simulink model "start_process_2018a"  (R2018a)
settings: Solver=FixedStepAuto  StartTime=0.0  StopTime=0.001  RelTol=1e-3
values from neighbouring files (symbols this model uses):
  trigger = true    [final_test.m]    (also in main_file.m; vel_measurement_final.m)
  velo = v_m * 1000    [final_test.m]
libraries: TcAdsLib x4
settings Model: Creator=chijiang  LastModifiedBy=chduan
settings OptimizationCC: LocalBlockOutputs=off
settings SFSimCC: SimUseLocalCustomCode=on
settings RTWCC: SystemTargetFile=TwinCAT.tlc  MakeCommand=make_tct  TemplateMakefile=tct_msbuild.tmf  Description=TwinCAT Target  GenerateReport=on  RTWUseLocalCustomCode=on  TargetLang=C++
settings STFCustomTargetCC: TargetLangStandard=C++03 (ISO)  CompOptLevelCompliant=on  MATLABClassNameForMDSCustomization=Simulink.SoftwareTarget.TargetSpecificTriggerConfigurationBase  SystemTargetFile=TwinCAT.tlc

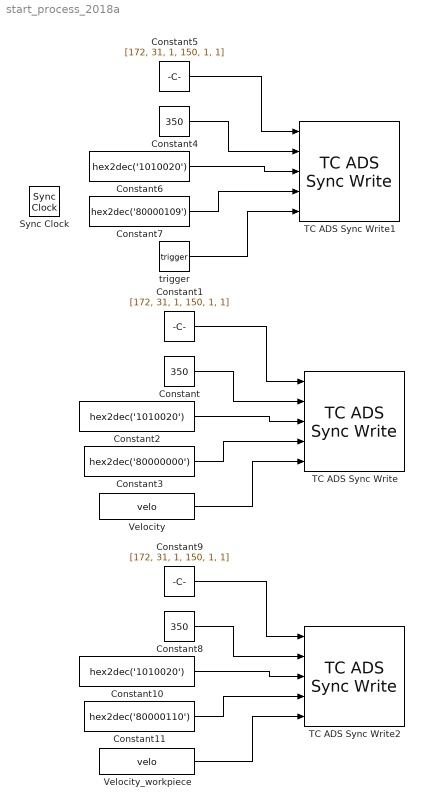
== system start_process_2018a ==
  Constant : Constant  Value=350  OutDataTypeStr=uint16
  Constant1 : Constant  Value=[172, 31, 1, 150, 1, 1]  OutDataTypeStr=uint8
  Constant10 : Constant  Value=hex2dec('1010020')  OutDataTypeStr=uint32
  Constant11 : Constant  Value=hex2dec('80000110')  OutDataTypeStr=uint32
  Constant2 : Constant  Value=hex2dec('1010020')  OutDataTypeStr=uint32
  Constant3 : Constant  Value=hex2dec('80000000')  OutDataTypeStr=uint32
  Constant4 : Constant  Value=350  OutDataTypeStr=uint16
  Constant5 : Constant  Value=[172, 31, 1, 150, 1, 1]  OutDataTypeStr=uint8
  Constant6 : Constant  Value=hex2dec('1010020')  OutDataTypeStr=uint32
  Constant7 : Constant  Value=hex2dec('80000109')  OutDataTypeStr=uint32
  Constant8 : Constant  Value=350  OutDataTypeStr=uint16
  Constant9 : Constant  Value=[172, 31, 1, 150, 1, 1]  OutDataTypeStr=uint8
  Sync Clock : TcAdsLib/Utilities/Sync Clock  OutputPortSelect=None  InputPortSelect=None
      settings: SourceProductName=Beckhoff TwinCAT ADS Interface
  TC ADS Sync Write : TcAdsLib/Synchronous/TC ADS Sync Write  SampleTime=-1  AbortSimulationOnAdsError=off  WriteDataType=double  WriteDataDim=1  WriteDataColToRowMajor=on  AdsTimeout=1  DirectFeedThrough=off  CreateSignalLabels=on  CodeGenConnectType=DataArea (OutputSrc)
      settings: SourceProductName=Beckhoff TwinCAT ADS Interface
  TC ADS Sync Write1 : TcAdsLib/Synchronous/TC ADS Sync Write  SampleTime=-1  AbortSimulationOnAdsError=off  WriteDataType=boolean  WriteDataDim=1  WriteDataColToRowMajor=on  AdsTimeout=1  DirectFeedThrough=off  CreateSignalLabels=on  CodeGenConnectType=DataArea (OutputSrc)
      settings: SourceProductName=Beckhoff TwinCAT ADS Interface
  TC ADS Sync Write2 : TcAdsLib/Synchronous/TC ADS Sync Write  SampleTime=-1  AbortSimulationOnAdsError=off  WriteDataType=double  WriteDataDim=1  WriteDataColToRowMajor=on  AdsTimeout=1  DirectFeedThrough=off  CreateSignalLabels=on  CodeGenConnectType=DataArea (OutputSrc)
      settings: SourceProductName=Beckhoff TwinCAT ADS Interface
  Velocity : Constant  Value=velo
  Velocity_workpiece : Constant  Value=velo
  trigger : Constant  Value=trigger  OutDataTypeStr=boolean
  wires:
  Constant/1 -> TC ADS Sync Write/2
  Constant2/1 -> TC ADS Sync Write/3
  Constant1/1 -> TC ADS Sync Write/1
  Velocity/1 -> TC ADS Sync Write/5
  Constant3/1 -> TC ADS Sync Write/4
  Constant7/1 -> TC ADS Sync Write1/4
  Constant4/1 -> TC ADS Sync Write1/2
  trigger/1 -> TC ADS Sync Write1/5
  Constant5/1 -> TC ADS Sync Write1/1
  Constant6/1 -> TC ADS Sync Write1/3
  Constant10/1 -> TC ADS Sync Write2/3
  Velocity_workpiece/1 -> TC ADS Sync Write2/5
  Constant9/1 -> TC ADS Sync Write2/1
  Constant11/1 -> TC ADS Sync Write2/4
  Constant8/1 -> TC ADS Sync Write2/2
